simulink model "pick_and_place_Linear_delta_robot"  (R2022b)
settings: Solver=ode23t  StartTime=0.0  StopTime=4  FixedStep=dt_solver  RelTol=1e-3  AbsTol=1e-3
model workspace (MAT data in the model file):
  Kd = 1.4
  Ki = 0
  Kp = 80
  dt_planner = 0.001
  dt_solver = 0.0002
values from neighbouring files (symbols this model uses):
  eeR = 0.02    [variables.m]
  q0 = [0.4447, 0.4447, 0.4447]    [variables.m]
  qd0 = [0 0 0]    [variables.m]
  R1 = 0.02    [variables.m]
  R2 = 0.015    [variables.m]
  Rbot = 0.036    [variables.m]
  Rtop = 0.364    [variables.m]
undefined symbols (not defined in the file or in its folder): entire, point1, point2, point3, X, Y, Z
libraries: sm_lib x60, nesl_utility x10, slpidlib x1
(part 3 of 3)

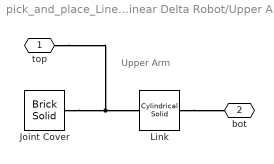
== system pick_and_place_Linear_delta_robot/Linear Delta Robot/Upper Arm2 ==
  note: Upper Arm
  " Link" : sm_lib/Body Elements/Cylindrical Solid  GraphicAmbientColor=[0.15 0.15 0.15 1.0]  BasedOnType=Density  CenterOfMass=[0 0 0]  CenterOfMassUnits=m  GraphicDiffuseColor=[0.8 0.8 0.8]  CylinderLength=L1  CylinderLengthUnits=m  CylinderRadius=R1  CylinderRadiusUnits=m  Density=1000  DensityUnits=kg/m^3  DoExposeReferenceFrame=off  GraphicEmissiveColor=[0.0 0.0 0.0 1.0]  ExportEntireGeometry=off  SerializedFrames=<Frames><Frame><Id>Frame1</Id><Value><Name>top</Name><Origin><Source>GeometricFeature</Source><FeatureName>top surface</FeatureName></Origin><PrimaryAxis><DefinedDirection>+X</DefinedDirection><Source>ReferenceFrame</Source><SourceDirection>-Z</SourceDirection><FeatureName></FeatureName></PrimaryAxis><SecondaryAxis><DefinedDirection>+Y</DefinedDirection><Source>ReferenceFrame</Source><SourceDirection>+X</SourceDirection><FeatureName></FeatureName></SecondaryAxis></Value></Frame><Frame><Id>Frame2</Id><Value><Name>bot</Name><Origin><Source>GeometricFeature</Source><FeatureName>top surface</FeatureName></Origin><PrimaryAxis><DefinedDirection>+Z</DefinedDirection><Source>ReferenceFrame</Source><SourceDirection>-Z</SourceDirection><FeatureName></FeatureName></PrimaryAxis><SecondaryAxis><DefinedDirection>+Y</DefinedDirection><Source>ReferenceFrame</Source><SourceDirection>+X</SourceDirection><FeatureName></FeatureName></SecondaryAxis></Value></Frame></Frames>  MarkerShape=Sphere  MarkerSize=10  GraphicType=FromGeometry  InertiaType=CalculateFromGeometry  Mass=1  MassUnits=kg  MomentsOfInertia=[1 1 1]  MomentsOfInertiaUnits=kg*m^2  GraphicOpacity=1.0  ProductsOfInertia=[0 0 0]  ProductsOfInertiaUnits=kg*m^2  GraphicShininess=75  GraphicSpecularColor=[0.5 0.5 0.5 1.0]  GraphicVisPropType=SimpleVisualProperties
  Joint Cover : sm_lib/Body Elements/Brick Solid  GraphicAmbientColor=[0.15 0.15 0.15 1.0]  BasedOnType=Density  BrickDimensions=[4*R1 6*R1 4*R1]  BrickDimensionUnits=m  CenterOfMass=[0 0 0]  CenterOfMassUnits=m  GraphicDiffuseColor=[0.5 0.5 0.5]  Density=1000  DensityUnits=kg/m^3  DoExposeReferenceFrame=on  GraphicEmissiveColor=[0.0 0.0 0.0 1.0]  ExportEntireGeometry=off  SerializedFrames=<Frames/>  MarkerShape=Sphere  MarkerSize=10  GraphicType=FromGeometry  InertiaType=CalculateFromGeometry  Mass=1  MassUnits=kg  MomentsOfInertia=[1 1 1]  MomentsOfInertiaUnits=kg*m^2  GraphicOpacity=1.0  ProductsOfInertia=[0 0 0]  ProductsOfInertiaUnits=kg*m^2  GraphicShininess=75  GraphicSpecularColor=[0.5 0.5 0.5 1.0]  GraphicVisPropType=SimpleVisualProperties
  top : PMIOPort  Side=Left
  bot : PMIOPort  Port=2  Side=Right
  connections:
  Joint Cover/RConn1 -- " Link"/LConn1 -- top/RConn1
  " Link"/RConn1 -- bot/RConn1

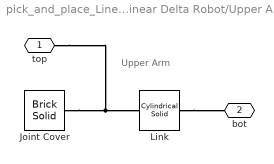
== system pick_and_place_Linear_delta_robot/Linear Delta Robot/Upper Arm3 ==
  note: Upper Arm
  " Link" : sm_lib/Body Elements/Cylindrical Solid  GraphicAmbientColor=[0.15 0.15 0.15 1.0]  BasedOnType=Density  CenterOfMass=[0 0 0]  CenterOfMassUnits=m  GraphicDiffuseColor=[0.8 0.8 0.8]  CylinderLength=L1  CylinderLengthUnits=m  CylinderRadius=R1  CylinderRadiusUnits=m  Density=1000  DensityUnits=kg/m^3  DoExposeReferenceFrame=off  GraphicEmissiveColor=[0.0 0.0 0.0 1.0]  ExportEntireGeometry=off  SerializedFrames=<Frames><Frame><Id>Frame1</Id><Value><Name>top</Name><Origin><Source>GeometricFeature</Source><FeatureName>top surface</FeatureName></Origin><PrimaryAxis><DefinedDirection>+X</DefinedDirection><Source>ReferenceFrame</Source><SourceDirection>-Z</SourceDirection><FeatureName></FeatureName></PrimaryAxis><SecondaryAxis><DefinedDirection>+Y</DefinedDirection><Source>ReferenceFrame</Source><SourceDirection>+X</SourceDirection><FeatureName></FeatureName></SecondaryAxis></Value></Frame><Frame><Id>Frame2</Id><Value><Name>bot</Name><Origin><Source>GeometricFeature</Source><FeatureName>top surface</FeatureName></Origin><PrimaryAxis><DefinedDirection>+Z</DefinedDirection><Source>ReferenceFrame</Source><SourceDirection>-Z</SourceDirection><FeatureName></FeatureName></PrimaryAxis><SecondaryAxis><DefinedDirection>+Y</DefinedDirection><Source>ReferenceFrame</Source><SourceDirection>+X</SourceDirection><FeatureName></FeatureName></SecondaryAxis></Value></Frame></Frames>  MarkerShape=Sphere  MarkerSize=10  GraphicType=FromGeometry  InertiaType=CalculateFromGeometry  Mass=1  MassUnits=kg  MomentsOfInertia=[1 1 1]  MomentsOfInertiaUnits=kg*m^2  GraphicOpacity=1.0  ProductsOfInertia=[0 0 0]  ProductsOfInertiaUnits=kg*m^2  GraphicShininess=75  GraphicSpecularColor=[0.5 0.5 0.5 1.0]  GraphicVisPropType=SimpleVisualProperties
  Joint Cover : sm_lib/Body Elements/Brick Solid  GraphicAmbientColor=[0.15 0.15 0.15 1.0]  BasedOnType=Density  BrickDimensions=[4*R1 6*R1 4*R1]  BrickDimensionUnits=m  CenterOfMass=[0 0 0]  CenterOfMassUnits=m  GraphicDiffuseColor=[0.5 0.5 0.5]  Density=1000  DensityUnits=kg/m^3  DoExposeReferenceFrame=on  GraphicEmissiveColor=[0.0 0.0 0.0 1.0]  ExportEntireGeometry=off  SerializedFrames=<Frames/>  MarkerShape=Sphere  MarkerSize=10  GraphicType=FromGeometry  InertiaType=CalculateFromGeometry  Mass=1  MassUnits=kg  MomentsOfInertia=[1 1 1]  MomentsOfInertiaUnits=kg*m^2  GraphicOpacity=1.0  ProductsOfInertia=[0 0 0]  ProductsOfInertiaUnits=kg*m^2  GraphicShininess=75  GraphicSpecularColor=[0.5 0.5 0.5 1.0]  GraphicVisPropType=SimpleVisualProperties
  top : PMIOPort  Side=Left
  bot : PMIOPort  Port=2  Side=Right
  connections:
  " Link"/RConn1 -- bot/RConn1
  top/RConn1 -- " Link"/LConn1 -- Joint Cover/RConn1

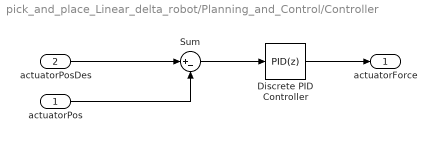
== system pick_and_place_Linear_delta_robot/Planning_and_Control/Controller ==
  actuatorPos : Inport
  actuatorPosDes : Inport  Port=2
  Discrete PID Controller : slpidlib/PID Controller  Controller=PID  Form=Parallel  TimeDomain=Discrete-time  UseExternalTs=off  SampleTime=-1  IntegratorMethod=Forward Euler  FilterMethod=Forward Euler  ControllerParametersSource=internal  P=P  I=I  UseKiTs=off  D=D  N=100  UseFilter=on  TunerSelectOption=Transfer Function Based (PID Tuner App)  InitialConditionSource=internal  InitialConditionForIntegrator=0  InitialConditionForFilter=0  DifferentiatorICPrevScaledInput=0  ExternalReset=none  TrackingMode=off  Kt=1  LimitOutput=off  SatLimitsSource=internal  UpperSaturationLimit=inf  LowerSaturationLimit=-inf  LinearizeAsGain=off  AntiWindupMode=none  Kb=1  LimitIntegrator=off  UpperIntegratorSaturationLimit=inf  LowerIntegratorSaturationLimit=-inf  POutMin=[]  POutMax=[]  IOutMin=[]  IOutMax=[]  DOutMin=[]  DOutMax=[]  NOutMin=[]  NOutMax=[]  SumOutMin=[]  SumOutMax=[]  SaturationOutMin=[]  SaturationOutMax=[]  PParamMin=[]  PParamMax=[]  IParamMin=[]  IParamMax=[]  DParamMin=[]  DParamMax=[]  NParamMin=[]  NParamMax=[]  KbParamMin=[]  KbParamMax=[]  KtParamMin=[]  KtParamMax=[]  KbOutMin=[]  KbOutMax=[]  KtOutMin=[]  KtOutMax=[]  IntegratorOutMin=[]  IntegratorOutMax=[]  FilterOutMin=[]  FilterOutMax=[]  SumI1OutMin=[]  SumI1OutMax=[]  SumI2OutMin=[]  SumI2OutMax=[]  SumI3OutMin=[]  SumI3OutMax=[]  SumI4OutMin=[]  SumI4OutMax=[]  SumDOutMin=[]  SumDOutMax=[]  DifferentiatorOutMin=[]  DifferentiatorOutMax=[]  FilterDiffOutCoefMin=[]  FilterDiffOutCoefMax=[]  ReciprocalOutMin=[]  ReciprocalOutMax=[]  SumDenOutMin=[]  SumDenOutMax=[]  SumNumOutMin=[]  SumNumOutMax=[]  DivideOutMin=[]  DivideOutMax=[]  UdiffTsProdOutMin=[]  UdiffTsProdOutMax=[]  NTsProdOutMin=[]  NTsProdOutMax=[]  UintegralTsProdOutMin=[]  UintegralTsProdOutMax=[]  UngainTsProdOutMin=[]  UngainTsProdOutMax=[]  ClampingZeroOutDataTypeStr=Inherit: Inherit via back propagation  ClampingZeroOutMin=[]  ClampingZeroOutMax=[]  FilterDenConstantOutDataTypeStr=Inherit: Inherit via back propagation  FilterDenConstantOutMin=[]  FilterDenConstantOutMax=[]  PCopyOutDataTypeStr=Inherit: Inherit via back propagation  PCopyOutMin=[]  PCopyOutMax=[]  NCopyOutDataTypeStr=Inherit: Inherit via back propagation  NCopyOutMin=[]  NCopyOutMax=[]  IntegratorContinuousStateAttributes=''  IntegratorStateMustResolveToSignalObject=off  IntegratorRTWStateStorageClass=Auto  FilterContinuousStateAttributes=''  FilterStateMustResolveToSignalObject=off  FilterRTWStateStorageClass=Auto  ParallelPVariant=InternalParameters  IdealPVariant=Disabled  IVariant=InternalParameters  DVariant=InternalParameters  IntegratorVariant=Discrete  SatVariant=Disabled  AWVariant=Passthrough  PCopyVariant=Disabled  TRVariant=Disabled  FdbkBlocksVariant=Forward  IdealPFdbkVariant=Disabled  SatFdbkVariant=Disabled  DerivativeFilterVariant=ForwardEulerFilter  NVariant=InternalParameters  NCopyVariant=Disabled  FilterICVariant=InternalICsFilter  IntegratorICVariant=InternalICs  ExternalResetVariant=Disabled  TRSumVariant=Passthrough  SumFdbkVariant=Disabled  SumVariant=Sum_PID  TsampFilterVariant=InternalTs  TsampNgainVariant=Passthrough  TsampIntegralVariant=Passthrough  ExternalSaturationOutDataTypeStr=Inherit: Same as second input
  Sum : Sum  Inputs=|+-
  actuatorForce : Outport
  wires:
  actuatorPosDes/1 -> Sum/1
  actuatorPos/1 -> Sum/2
  Sum/1 -> Discrete PID Controller/1
  Discrete PID Controller/1 -> actuatorForce/1

== matlab function pick_and_place_Linear_delta_robot/Planning_and_Control/Path Planner ==
  data: eePos input size=3; eePosDes output size=3; eeVelDes output; eeVel input size=3; t input size=1; currentMode output size=1
function [eePosDes, eeVelDes, currentMode] = Planner(eePos, eeVel, t)
%% Pour IHM 
%function [eePosDes, eeVelDes, currentMode] = Planner(eePos, eeVel, t, TrajectoryType)%% bedelth juste pour IHM


% ============================================================
% SIMPLE TRAJECTORY PLANNER
% LINEAR DELTA ROBOT
% TRAJECTORY TYPES:
% 0 -> Circular trajectory
% 1 -> Rectangular trajectory
% 2 -> Point-to-Point trajectory
%3-> test 1 fixe 
% ============================================================

%% ===========================================================
% SELECT TRAJECTORY
%% ===========================================================
trajectoryType = 0;

%% pour IHM 
%trajectoryType = TrajectoryType; % zitha juste pour ihm 
currentMode = trajectoryType;





%% ===========================================================
% PERSISTENT VARIABLES
%% ===========================================================
persistent plan currentTarget
if isempty(plan)
    plan = true;
    currentTarget = [ ...
        -0.08;
        -0.08;
        -0.35];
end
%% ===========================================================
% WORKSPACE CENTER
%% ===========================================================
xc = 0.0;
yc = 0.0;
zc = -0.35;
%% ===========================================================
% TRAJECTORY PARAMETERS
%% ===========================================================

%%%%%%%%%%%% cercle horizontal centré sur : (0, 0, −0.35)
%%%%%%%%%%%  w = omega permet de ralentir ou accélérer  ω=2πf
radius = 0.01;
%omega  = 2*pi*0.05;avec time=3 on peut voir que 15% de cercle 
omega = 2*pi*(1/3);

rectWidth  = 0.12;
rectHeight = 0.08;
rectSpeed  = 0.10;
%% ===========================================================
% TRAJECTORY GENERATION
%% ===========================================================
switch trajectoryType
    %% =======================================================
    % CIRCULAR TRAJECTORY
    %% =======================================================
    case 0
       
             % =========================================
            % WAIT BEFORE STARTING CIRCLE
            % =========================================      
           t_delay = 1.0;       
            if t < t_delay        
                x = xc + radius;
                y = yc;
                z = zc;
        
              vx = 0;
                vy = 0;
               vz = 0;        
            else
               tau = t - t_delay; 
               x = xc + radius*cos(omega*tau);
                y = yc + radius*sin(omega*tau);
             % y = yc + radius*sin(omega*t);
                z = zc;

               vx = -radius*omega*sin(omega*tau);
               vy =  radius*omega*cos(omega*tau);
               vz = 0;
            end
            eePosDes = [x; y; z];
            eeVelDes = [vx; vy; vz];
    

   

%% =======================================================
% RECTANGULAR TRAJECTORY V3
% RECTANGLE + ROUNDED CORNERS + SMOOTH STARTUP
%% =======================================================
case 1

    %% ===================================================
    % PARAMETERS
    %% ===================================================

    currentMode = 1;

    % Stabilization
    t_delay = 0.5;

    % Rectangle dimensions
    rectWidth  = 0.04;     % 4 cm
    rectHeight = 0.03;     % 3 cm

    % Motion speed
    rectSpeed = 0.04;
    

    % Rounded corner radius
    rCorner = 0.005;

    %% ===================================================
    % RECTANGLE LIMITS
    %% ===================================================

    x0 = xc - rectWidth/2;
    x1 = xc + rectWidth/2;

    y0 = yc - rectHeight/2;
    y1 = yc + rectHeight/2;

    %% ===================================================
    % USEFUL LIMITS
    %% ===================================================

    xL = x0 + rCorner;
    xR = x1 - rCorner;

    yB = y0 + rCorner;
    yT = y1 - rCorner;

    %% ===================================================
    % SEGMENT TIMES
    %% ===================================================

    Lx = rectWidth  - 2*rCorner;
    Ly = rectHeight - 2*rCorner;

    TlineX = Lx / rectSpeed;
    TlineY = Ly / rectSpeed;

    Tarc = (pi/2)*rCorner / rectSpeed;

    totalTime = ...
        2*TlineX + ...
        2*TlineY + ...
        4*Tarc;

    %% ===================================================
    % SMOOTH STARTUP
    %% ===================================================

    if t < t_delay

        r = t / t_delay;

        % Quintic interpolation
        s = 10*r^3 - 15*r^4 + 6*r^5;

        % Quintic derivative
        ds = (30*r^2 - 60*r^3 + 30*r^4)/t_delay;

        % Initial position
        p0 = [0;0;zc];

        % First trajectory point
        p1 = [xL;y0;zc];

        % Position
        eePosDes = p0 + s*(p1-p0);

        % Velocity continuity
        vTarget = [rectSpeed;0;0];

        eeVelDes = ds*(p1-p0) + s*vTarget;

        return;

    end

    %% ===================================================
    % RECTANGLE MOTION
    %% ===================================================
    t_rect = t - t_delay;
    tau = mod(t_rect,totalTime);
    %% ===================================================
    % SEGMENT 1 : BOTTOM
    %% ===================================================
    if tau < TlineX
        s = tau;
        x = xL + rectSpeed*s;
        y = y0;
        vx = rectSpeed;
        vy = 0;
    %% ===================================================
    % ARC 1 : BOTTOM RIGHT
    %% ===================================================
    elseif tau < TlineX + Tarc
        s = tau - TlineX;
        theta = -pi/2 + (rectSpeed/rCorner)*s;
        x = xR + rCorner*cos(theta);
        y = yB + rCorner*sin(theta);
        vx = -rectSpeed*sin(theta);
        vy =  rectSpeed*cos(theta);
    %% ===================================================
    % SEGMENT 2 : RIGHT
    %% ===================================================
    elseif tau < TlineX + Tarc + TlineY
        s = tau - TlineX - Tarc;
        x = x1;
        y = yB + rectSpeed*s;
        vx = 0;
        vy = rectSpeed;
    %% ===================================================
    % ARC 2 : TOP RIGHT
    %% ===================================================
    elseif tau < TlineX + Tarc + TlineY + Tarc
        s = tau - TlineX - Tarc - TlineY;
        theta = 0 + (rectSpeed/rCorner)*s;
        x = xR + rCorner*cos(theta);
        y = yT + rCorner*sin(theta);
        vx = -rectSpeed*sin(theta);
        vy =  rectSpeed*cos(theta);
    %% ===================================================
    % SEGMENT 3 : TOP
    %% ===================================================
    elseif tau < 2*TlineX + 2*Tarc + TlineY
        s = tau - TlineX - 2*Tarc - TlineY;
        x = xR - rectSpeed*s;
        y = y1;
        vx = -rectSpeed;
        vy = 0;
    %% ===================================================
    % ARC 3 : TOP LEFT
    %% ===================================================
    elseif tau < 2*TlineX + 3*Tarc + TlineY
        s = tau - 2*TlineX - 2*Tarc - TlineY;
        theta = pi/2 + (rectSpeed/rCorner)*s;
        x = xL + rCorner*cos(theta);
        y = yT + rCorner*sin(theta);
        vx = -rectSpeed*sin(theta);
        vy =  rectSpeed*cos(theta);
    %% ===================================================
    % SEGMENT 4 : LEFT
    %% ===================================================
    elseif tau < 2*TlineX + 3*Tarc + 2*TlineY
        s = tau - 2*TlineX - 3*Tarc - TlineY;
        x = x0;
        y = yT - rectSpeed*s;
        vx = 0;
        vy = -rectSpeed;
    %% ===================================================
    % ARC 4 : BOTTOM LEFT
    %% ===================================================
    else
        s = tau - 2*TlineX - 3*Tarc - 2*TlineY;
        theta = pi + (rectSpeed/rCorner)*s;
        x = xL + rCorner*cos(theta);
        y = yB + rCorner*sin(theta);
        vx = -rectSpeed*sin(theta);
        vy =  rectSpeed*cos(theta);
    end
    %% ===================================================
    % OUTPUT
    %% ===================================================
    z = zc;
    eePosDes = [x;y;z];
    eeVelDes = [vx;vy;0];



    %% =======================================================
    % POINT TO POINT TRAJECTORY
    %% =======================================================
    case 2    
    
        % Paramètres des directions de départ et d'arrivée (true ou false)
        startVertical = false; 
        endVertical   = false;
        
        % Appel de la fonction de planification par polynômes
        [eePosDes, eeVelDes, done] = gotoPosition( ...
            currentTarget, ...
            eePos, ...
            eeVel, ...
            t, ...
            startVertical, ...
            endVertical, ...
            plan);
        
        % Une fois la planification initiale faite au temps t0, 
        % on passe 'plan' à false pour ne pas recalculer le polynôme à chaque pas de temps
        if plan
            plan = false;
        end
        
        % Optionnel : Si le robot est arrivé à destination, on peut changer de cible 
        % ou simplement arrêter. Ici il s'arrête à la cible.
        if done
            % Robot arrivé au point
        end



    %%%%%%%%%%%%%%%%%%%%%%%%%%%%%%%%%%%%%%%%%%%%%%%%%%%%%%%%%%%%%%%%%%%%%%%
    % case 3 nouveau 
    %%%%%%%%%%%%%%%%%%%%%%%%%%%%%%%%%%%%%%%%%%%%%%%%%%%%%%%%%%%%%%%%%%%%%%%%
    case 3
        % =====================================================
        % FIXED POINT TEST
        % =====================================================
        eePosDes = [
             0.00;
             0.00;
            -0.35
        ];
    
        eeVelDes = [
            0;
            0;
            0
        ];
    


    %% =======================================================
    % DEFAULT
    %% =======================================================
    otherwise
        eePosDes = [xc; yc; zc];
        eeVelDes = [0;0;0];
end

end



%% ===========================================================
% GOTO POSITION
%% ===========================================================

function [eePosDes, eeVelDes, done] = gotoPosition( ...
    eePosGoal, ...
    eePos, ...
    eeVel, ...
    t, ...
    startVertical, ...
    endVertical, ...
    plan)

if startVertical
    startDirectionGoal = [0;0;-0.2];
else
    startDirectionGoal = eeVel;
end
if endVertical
    endDirectionGoal = [0;0;0.2];
else
    endDirectionGoal = [0;0;0];
end
timeToGoal = 1.0;
[eePosDes, eeVelDes, atGoal] = gotoGoal( ...
    plan, ...
    t, ...
    timeToGoal, ...
    eePos, ...
    eeVel, ...
    eePosGoal, ...
    startDirectionGoal, ...
    endDirectionGoal);
done = atGoal;
end

%% ===========================================================
% GOTO GOAL
%% ===========================================================

function [eePosDes, eeVelDes, atGoal] = gotoGoal( ...
    plan, ...
    t, ...
    timeToGoal, ...
    eePos, ...
    eeVel, ...
    eePosGoal, ...
    startDirectionGoal, ...
    endDirectionGoal)

persistent cpoly cdpoly spoly sdpoly t0 tf

if isempty(tf)
    cpoly  = zeros(3,4);
    cdpoly = zeros(3,3);
    spoly  = zeros(1,6);
    sdpoly = zeros(1,5);
    t0 = 0;
    tf = 0;
end

if plan
    t0 = t;
    tf = t0 + timeToGoal;
    [cpoly, cdpoly, spoly, sdpoly] = getTrajectory( ...
        t0, ...
        tf, ...
        eePos, ...
        eePosGoal, ...
        startDirectionGoal, ...
        endDirectionGoal);
end

t = min(t,tf);
s = polyval(spoly,t);
eePosDes = [ ...
    polyval(cpoly(1,:),s);
    polyval(cpoly(2,:),s);
    polyval(cpoly(3,:),s)];

eeVelDes = [ ...
    polyval(cdpoly(1,:),s);
    polyval(cdpoly(2,:),s);
    polyval(cdpoly(3,:),s)] * polyval(sdpoly,t);

errPos = norm(eePosGoal - eePos);
errVel = norm(eeVel);

atGoal = (errPos < 0.003) && (errVel < 0.01);
end

%% ===========================================================
% GET TRAJECTORY
%% ===========================================================

function [cpoly, cdpoly, spoly, sdpoly] = getTrajectory( ...
    t0, ...
    tf, ...
    eePos, ...
    eePosGoal, ...
    startDirectionGoal, ...
    endDirectionGoal)

cpoly  = zeros(3,4);
cdpoly = zeros(3,3);

for i = 1:3
    cpoly(i,:) = getPoly3( ...
        0, ...
        1, ...
        eePos(i), ...
        startDirectionGoal(i), ...
        eePosGoal(i), ...
        endDirectionGoal(i));
    pd = polyder(cpoly(i,:));
    if length(pd) == 3
        cdpoly(i,:) = pd;
    else
        cdpoly(i,:) = [0 0 0];
    end
end

spoly = getPoly5( ...
    t0, ...
    tf, ...
    0,0,0, ...
    1,0,0);
sdpoly = polyder(spoly);
end

%% ===========================================================
% POLYNOMIAL ORDER 3
%% ===========================================================

function p = getPoly3( ...
    t0, ...
    tf, ...
    x0, ...
    v0, ...
    xf, ...
    vf)

A = [ ...
    t0^3    t0^2   t0   1;
    3*t0^2  2*t0   1    0;
    tf^3    tf^2   tf   1;
    3*tf^2  2*tf   1    0];

b = [x0;v0;xf;vf];

p = A\b;

end

%% ===========================================================
% POLYNOMIAL ORDER 5
%% ===========================================================

function p = getPoly5( ...
    t0, ...
    tf, ...
    x0, ...
    v0, ...
    a0, ...
    xf, ...
    vf, ...
    af)

A = [ ...
    t0^5      t0^4      t0^3    t0^2   t0   1;
    5*t0^4    4*t0^3    3*t0^2  2*t0  1    0;
    20*t0^3   12*t0^2   6*t0    2     0    0;
    tf^5      tf^4      tf^3    tf^2   tf   1;
    5*tf^4    4*tf^3    3*tf^2  2*tf  1    0;
    20*tf^3   12*tf^2   6*tf    2     0    0];

b = [x0;v0;a0;xf;vf;af];

p = A\b;

end

== matlab function pick_and_place_Linear_delta_robot/Planning_and_Control/Forward Kinematics ==
  data: actuatorPos input size=3; eePos output size=3; actuatorVel input size=3; eeVel output
%function [eePos, eeVel] = FK(actuatorPos, actuatorVel)
% Wrapper around sm_pick_and_place_fk.m, which creates a persistent
% KinematicsSolver object for the forwards kinematics problem and then
% solves it.
%%%%% coder.extrinsic('analytic_linear_delta_robot_fk');
%persistent init
%if isempty(init)
   % init = true;
   % eePos = zeros(3,1);
  %  eeVel = zeros(3,1);
 %   status = 1;
%end
%[eePos, eeVel, status] = analytic_linear_delta_robot_fk(actuatorPos, actuatorVel);
%if status ~= 1
 %   error('fk solve failed')
%end
%_________________________________________
%function [eePos, eeVel] = FK(actuatorPos, actuatorVel)
%persistent init
%if isempty(init)
%    init = true;
%end
%[eePos, eeVel, status] = ...
%    analytic_linear_delta_robot_fk(actuatorPos, actuatorVel);
%if status ~= 1
%    eePos = [0;0;-0.35];
%    eeVel = [0;0;0];
%end
%end
%________________________________________
function [eePos, eeVel] = fK(actuatorPos, actuatorVel)
persistent lastPos lastVel
if isempty(lastPos)
    lastPos = [0;0;-0.35];
    lastVel = [0;0;0];
end
[eePosTemp, eeVelTemp, status] = fk(actuatorPos, actuatorVel);

if status == 1
    eePos = eePosTemp;
    eeVel = eeVelTemp;
    lastPos = eePosTemp;
    lastVel = eeVelTemp;
else
    eePos = lastPos;
    eeVel = lastVel;
end
end

== matlab function pick_and_place_Linear_delta_robot/Planning_and_Control/Inverse Kinematics ==
  data: eePosDes input size=3; actuatorPosDes output size=3
function actuatorPosDes = IK(eePosDes)
% ============================================================
% INVERSE KINEMATICS WRAPPER
% ============================================================
%coder.extrinsic('analytic_linear_delta_robot_ik');
persistent lastValidPos
if isempty(lastValidPos)
    %lastValidPos = [0.2;0.2;0.2];
    lastValidPos = [0.4447;0.4447;0.4447];
end
% ============================================================
% PREALLOCATION
% ============================================================
actuatorPosDesTemp = zeros(3,1);
status = 0;
% ============================================================
% CALL IK
% ============================================================
[actuatorPosDesTemp, status] = ik(eePosDes);
% ============================================================
% SAFETY
% ============================================================
status = double(status);
% ============================================================
% VALID SOLUTION
% ============================================================
if status == 1
    actuatorPosDes = actuatorPosDesTemp;
    lastValidPos = actuatorPosDesTemp;
else
  %------bech ne7i msg erreur :  disp('IK failed -> keeping last valid position');
    actuatorPosDes = lastValidPos;
end
end
